simulink model "nonlinear_seesaw_matlabsimulink_29_04_2024"  (R2023b)
settings: Solver=VariableStepAuto  StartTime=0.0  StopTime=3  RelTol=1e-3
values from neighbouring files (symbols this model uses):
  g = 9.81    [nonlinear_seesaw_matlabsimulink_29_04_2024_inizalise.m]
  h = 0.1    [nonlinear_seesaw_matlabsimulink_29_04_2024_inizalise.m]
  Jconst = mf*h^2+Jb    (= 0.501)    [nonlinear_seesaw_matlabsimulink_29_04_2024_inizalise.m]
  mf = 0.1    [nonlinear_seesaw_matlabsimulink_29_04_2024_inizalise.m]
settings Model: Creator=dmplab  LastModifiedBy=Krish
settings DebuggingCC: UnconnectedInputMsg=warning  UnconnectedOutputMsg=warning  UnconnectedLineMsg=warning
settings ModelReferenceCC: EnableRefExpFcnMdlSchedulingChecks=on
settings RTWCC: DLArmComputeVersion=19.05

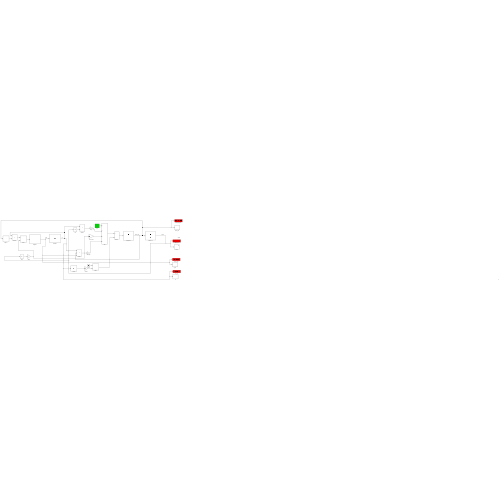
[thumbnail: Simulink's stored preview of the top-level diagram]
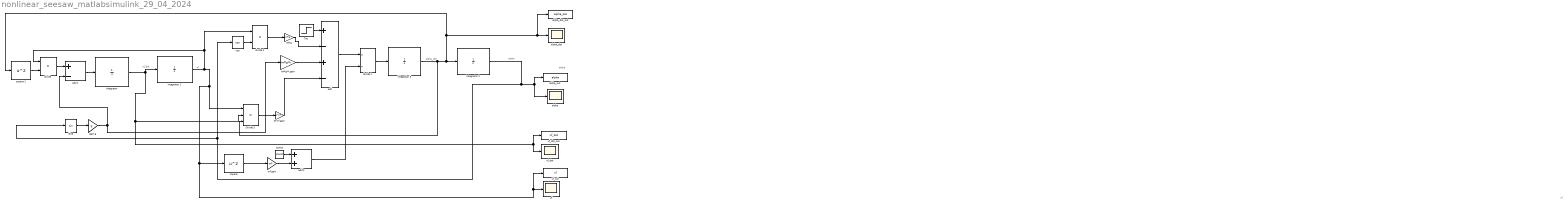
== system nonlinear_seesaw_matlabsimulink_29_04_2024 ==
  note: alpha_dot
  note: xf_dot
  note: xf
  note: alpha
  note: alpha
  note: xf
  2*mf gain : Gain  Gain=2*mf
  Divide 3 : Product  Inputs=***
  Integrator {,1..3} (4 alike) : Integrator
  Jconst : Constant  Value=Jconst
  Sine : Trigonometry
  Tau : Step  SampleTime=0
  add : Sum  Inputs=+-+-
  add 1 : Sum  Inputs=+-
  add 2 : Sum
  alpha : Scope
  alpha_dot : Scope
  alpha_dot_out : ToWorkspace  VariableName=alpha_dot  SaveFormat=Timeseries  SampleTime=-1
  alpha_out : ToWorkspace  VariableName=alpha  SaveFormat=Timeseries  SampleTime=-1
  cos : Trigonometry  Operator=cos
  divide : Product  Inputs=**
  divide 1 : Product  Inputs=*/
  divide 2 : Product  Inputs=**
  gain g : Gain  Gain=g
  mf gain : Gain  Gain=mf
  mf*g : Gain  Gain=mf*g
  mf*g*h gain : Gain  Gain=mf*g*h
  square : Math  Operator=square
  square 1 : Math  Operator=square
  xf : Scope
  xf_dot : Scope
  xf_dot_out : ToWorkspace  VariableName=xf_dot  SaveFormat=Timeseries  SampleTime=-1
  xf_out : ToWorkspace  VariableName=xf  SaveFormat=Timeseries  SampleTime=-1
  wires:
  "Integrator "/1 -> Integrator 1/1, xf_dot/1, xf_dot_out/1, Divide 3/2
  Integrator 3/1 -> Integrator 2/1, square 1/1, alpha_dot_out/1, alpha_dot/1, Divide 3/3
  add 1/1 -> "Integrator "/1
  Integrator 1/1 -> xf/1, xf_out/1, square/1, Divide 3/1, divide/1, divide 2/1
  divide/1 -> add 1/1
  Integrator 2/1 -> alpha_out/1, alpha/1, cos/1, Sine/1
  gain g/1 -> add 1/2, mf*g*h gain/1
  Sine/1 -> gain g/1
  square 1/1 -> divide/2
  Jconst/1 -> add 2/1
  mf gain/1 -> add 2/2
  square/1 -> mf gain/1
  add/1 -> divide 1/1
  divide 1/1 -> Integrator 3/1
  add 2/1 -> divide 1/2
  mf*g/1 -> add/2
  Tau/1 -> add/1
  divide 2/1 -> mf*g/1
  cos/1 -> divide 2/2
  mf*g*h gain/1 -> add/3
  2*mf gain/1 -> add/4
  Divide 3/1 -> 2*mf gain/1
